simulink model "UAVUGV3"  (R2018a)
settings: Solver=VariableStepAuto  StartTime=0.0  StopTime=300  RelTol=1e-3
libraries: simulink x2
settings Model: Creator=wangluo  LastModifiedBy=wangluo

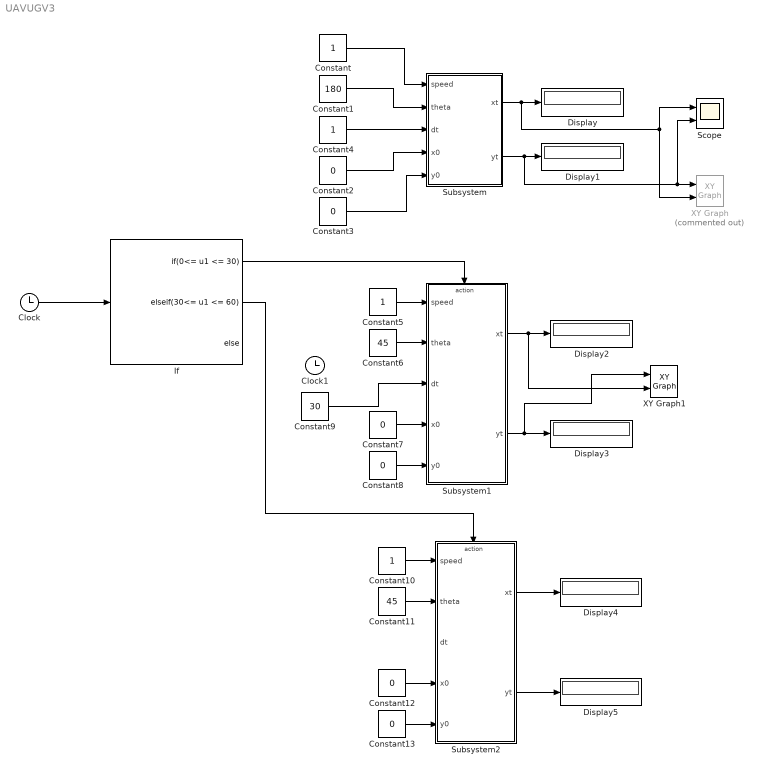
== system UAVUGV3 ==
  Clock : Clock
      settings: Decimation=300
  Clock1 : Clock
      settings: Decimation=3
  Constant{,4..5,10} (4 alike) : Constant
  Constant1 : Constant  Value=180
  Constant11 : Constant  Value=45
  Constant{2..3,7..8,12..13} (6 alike) : Constant  Value=0
  Constant6 : Constant  Value=45
  Constant9 : Constant  Value=30
  Display{,1..5} (6 alike) : Display
  If : If  IfExpression=0<= u1 <= 30  ElseIfExpressions=30<= u1 <= 60
  Scope : Scope  NumInputPorts=2
  Subsystem : Subsystem
  Subsystem1 : Subsystem
  Subsystem2 : Subsystem
  XY Graph : simulink/Sinks/XY Graph  Commented=on  xmin=-1  xmax=1  ymin=-1  ymax=1  st=-1
  XY Graph1 : simulink/Sinks/XY Graph  xmin=-100  xmax=200  ymin=-100  ymax=150  st=-1
  wires:
  Constant/1 -> Subsystem/1(speed)
  Constant1/1 -> Subsystem/2(theta)
  Constant2/1 -> Subsystem/4(x0)
  Constant3/1 -> Subsystem/5(y0)
  Constant4/1 -> Subsystem/3(dt)
  Subsystem/1(xt) -> XY Graph/2, Scope/1, Display/1
  Subsystem/2(yt) -> Scope/2, XY Graph/1, Display1/1
  If/1 -> Subsystem1/Action
  Constant5/1 -> Subsystem1/1(speed)
  Constant6/1 -> Subsystem1/2(theta)
  Constant7/1 -> Subsystem1/4(x0)
  Constant8/1 -> Subsystem1/5(y0)
  Subsystem1/1(xt) -> XY Graph1/2, Display2/1
  Subsystem1/2(yt) -> XY Graph1/1, Display3/1
  Clock/1 -> If/1
  Subsystem2/1(xt) -> Display4/1
  Subsystem2/2(yt) -> Display5/1
  Constant13/1 -> Subsystem2/5(y0)
  Constant11/1 -> Subsystem2/2(theta)
  ? -> Subsystem2/3(dt)
  Constant10/1 -> Subsystem2/1(speed)
  Constant12/1 -> Subsystem2/4(x0)
  If/2 -> Subsystem2/Action
  Constant9/1 -> Subsystem1/3(dt)

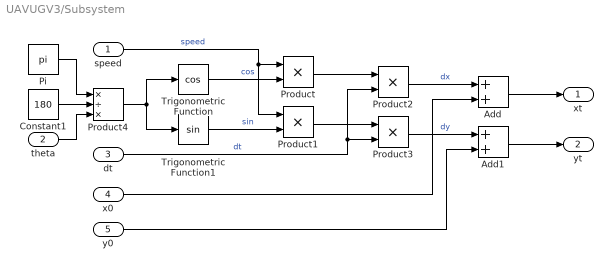
== system UAVUGV3/Subsystem ==
  speed : Inport
  theta : Inport  Port=2
  dt : Inport  Port=3
  x0 : Inport  Port=4
  y0 : Inport  Port=5
  Add : Sum
  Add1 : Sum
  Constant1 : Constant  Value=180
  Pi : Constant  Value=pi
  Product{,1..3} (4 alike) : Product
  Product4 : Product  Inputs=*/*
  Trigonometric Function : Trigonometry  Operator=cos
  Trigonometric Function1 : Trigonometry
  xt : Outport
  yt : Outport  Port=2
  wires:
  Add/1 -> xt/1
  Trigonometric Function/1 -> Product/2  "cos"
  y0/1 -> Add1/2
  Add1/1 -> yt/1
  Trigonometric Function1/1 -> Product1/2  "sin"
  x0/1 -> Add/2
  speed/1 -> Product1/1, Product/1  "speed"
  Product/1 -> Product2/1
  dt/1 -> Product2/2, Product3/2  "dt"
  Product2/1 -> Add/1  "dx"
  Product1/1 -> Product3/1
  Product3/1 -> Add1/1  "dy"
  Pi/1 -> Product4/1
  Constant1/1 -> Product4/2
  theta/1 -> Product4/3
  Product4/1 -> Trigonometric Function1/1, Trigonometric Function/1

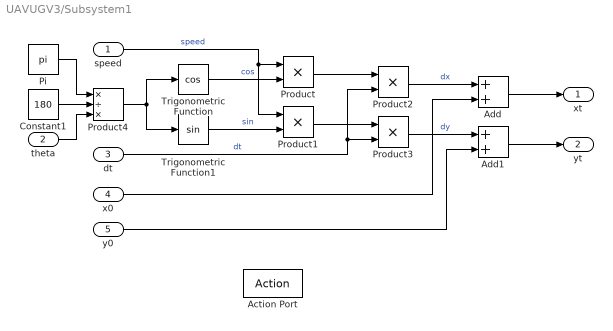
== system UAVUGV3/Subsystem1 ==
  speed : Inport
  theta : Inport  Port=2
  dt : Inport  Port=3
  x0 : Inport  Port=4
  y0 : Inport  Port=5
  Action Port : ActionPort  ActionType=then
  Add : Sum
  Add1 : Sum
  Constant1 : Constant  Value=180
  Pi : Constant  Value=pi
  Product{,1..3} (4 alike) : Product
  Product4 : Product  Inputs=*/*
  Trigonometric Function : Trigonometry  Operator=cos
  Trigonometric Function1 : Trigonometry
  xt : Outport
  yt : Outport  Port=2
  wires:
  Add/1 -> xt/1
  Trigonometric Function/1 -> Product/2  "cos"
  y0/1 -> Add1/2
  Add1/1 -> yt/1
  Trigonometric Function1/1 -> Product1/2  "sin"
  x0/1 -> Add/2
  speed/1 -> Product1/1, Product/1  "speed"
  Product/1 -> Product2/1
  dt/1 -> Product2/2, Product3/2  "dt"
  Product2/1 -> Add/1  "dx"
  Product1/1 -> Product3/1
  Product3/1 -> Add1/1  "dy"
  Pi/1 -> Product4/1
  Constant1/1 -> Product4/2
  theta/1 -> Product4/3
  Product4/1 -> Trigonometric Function1/1, Trigonometric Function/1

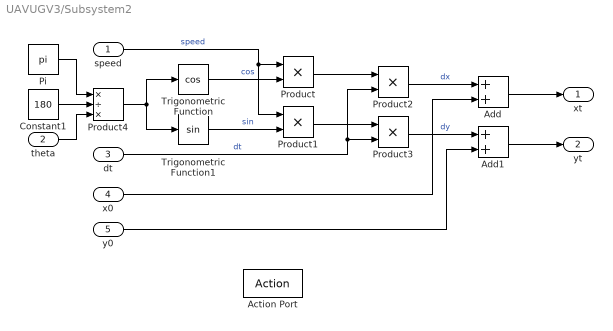
== system UAVUGV3/Subsystem2 ==
  speed : Inport
  theta : Inport  Port=2
  dt : Inport  Port=3
  x0 : Inport  Port=4
  y0 : Inport  Port=5
  Action Port : ActionPort  ActionType=elseif
  Add : Sum
  Add1 : Sum
  Constant1 : Constant  Value=180
  Pi : Constant  Value=pi
  Product{,1..3} (4 alike) : Product
  Product4 : Product  Inputs=*/*
  Trigonometric Function : Trigonometry  Operator=cos
  Trigonometric Function1 : Trigonometry
  xt : Outport
  yt : Outport  Port=2
  wires:
  Add/1 -> xt/1
  Trigonometric Function/1 -> Product/2  "cos"
  y0/1 -> Add1/2
  Add1/1 -> yt/1
  Trigonometric Function1/1 -> Product1/2  "sin"
  x0/1 -> Add/2
  speed/1 -> Product1/1, Product/1  "speed"
  Product/1 -> Product2/1
  dt/1 -> Product2/2, Product3/2  "dt"
  Product2/1 -> Add/1  "dx"
  Product1/1 -> Product3/1
  Product3/1 -> Add1/1  "dy"
  Pi/1 -> Product4/1
  Constant1/1 -> Product4/2
  theta/1 -> Product4/3
  Product4/1 -> Trigonometric Function1/1, Trigonometric Function/1
